simulink model "LQR_DE6000008"  (R2025b)
settings: Solver=VariableStepAuto  StartTime=0.0  StopTime=10.0  RelTol=1e-3
undefined symbols (not defined in the file or in its folder): A, B, K_LQR_i, K_LQR_x, m, n, r, x0_sylv
settings Model: Creator=salvo  LastModifiedBy=salvo

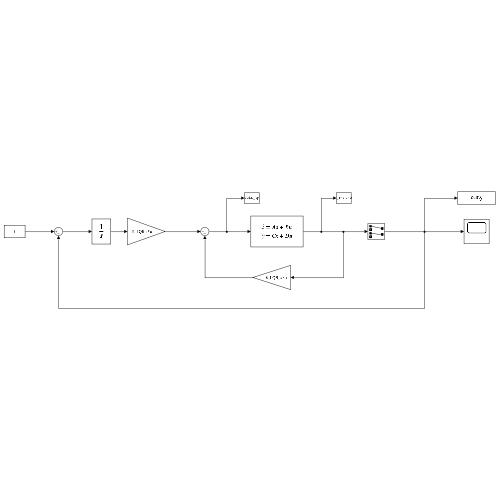
[thumbnail: Simulink's stored preview of the top-level diagram]
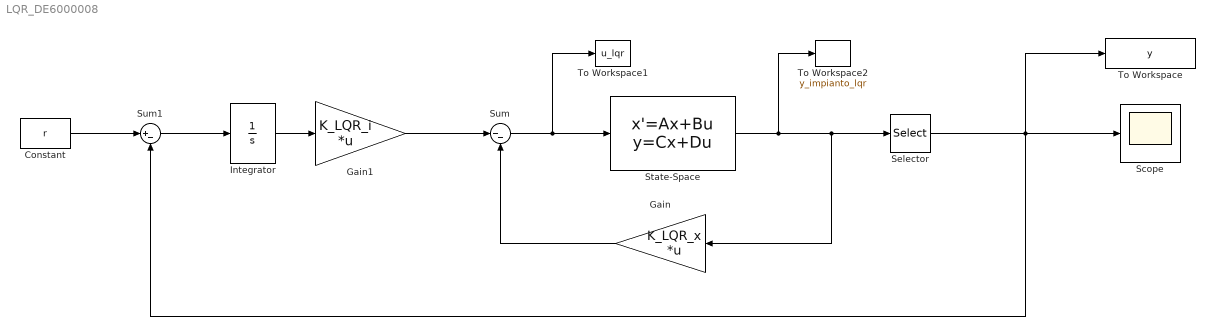
== system LQR_DE6000008 ==
  Constant : Constant  Value=r
  Gain : Gain  Gain=K_LQR_x  Multiplication=Matrix(K*u)
  Gain1 : Gain  Gain=K_LQR_i  Multiplication=Matrix(K*u)
  Integrator : Integrator
  Scope : Scope
      settings: ActiveDisplayYMinimum=-0.15571176263239439  ActiveDisplayYMaximum=0.25772573736760651
  Selector : Selector  InputPortWidth=4  IndexOptions=Index vector (dialog)  Indices=[1 3]  OutputSizes=1
  State-Space : StateSpace  A=A  B=B  C=eye(n)  D=zeros(n,m)  InitialCondition=x0_sylv
  Sum : Sum  Inputs=|--
  Sum1 : Sum  Inputs=|+-
  To Workspace : ToWorkspace  VariableName=y  SaveFormat=Timeseries  SampleTime=-1
  To Workspace1 : ToWorkspace  VariableName=u_lqr  SaveFormat=Timeseries  SampleTime=-1
  To Workspace2 : ToWorkspace  VariableName=y_impianto_lqr  SaveFormat=Timeseries  SampleTime=-1
  wires:
  Integrator/1 -> Gain1/1
  Gain/1 -> Sum/2
  Gain1/1 -> Sum/1
  Sum/1 -> To Workspace1/1, State-Space/1
  Sum1/1 -> Integrator/1
  State-Space/1 -> To Workspace2/1, Gain/1, Selector/1
  Selector/1 -> Scope/1, To Workspace/1, Sum1/2
  Constant/1 -> Sum1/1
